simulink model "A1_DC_coupled_AC_output_grid_interface_DC_forming"  (R2022b)
settings: Solver=ode4  StartTime=0.0  StopTime=tend  FixedStep=ts  RelTol=1e-3
values from neighbouring files (symbols this model uses):
  C = 80000e-6    (= 0.08)    [A1_Parameters.m]
  C_bc_ESS = C_bc_ESS    (= 0.005)    [A1_Parameters.m]
  C_bc_PV = C_bc_PV    (= 0.005)    [A1_Parameters.m]
  C_bc_SC = C_bc_SC    (= 0.005)    [A1_Parameters.m]
  C_SC_set = C_SC * Vdc_SCunit^2/Vdc_SC^2    (= 0.617283950617)    [A1_Parameters.m]
  Cf = 0.08    [A1_Parameters.m]
  f0 = 60    [A1_Parameters.m]
  fc = 20    [A1_Parameters.m]
  fc1 = 1000    [A1_Parameters.m]
  fv = 100    [A1_Parameters.m]
  Idcbase = Sbase/Vdc_nom    (= 1250)    [A1_Parameters.m]
  J = [0 -1; 1 0]    [A1_Parameters.m]
  Ki_c = 500    [A1_Parameters.m]
  Ki_v = 500    [A1_Parameters.m]
  Ki_v1 = 1000    [A1_Parameters.m]
  Kp_c = 10    [A1_Parameters.m]
  Kp_v = 5    [A1_Parameters.m]
  Kp_v1 = 50    [A1_Parameters.m]
  L_bc_ESS = 4e-4    (= 0.0004)    [A1_Parameters.m]
  L_bc_PV = 4e-4    (= 0.0004)    [A1_Parameters.m]
  L_bc_SC = 4e-4    (= 0.0004)    [A1_Parameters.m]
  Lf = 0.10    (= 0.1)    [A1_Parameters.m]
  Pset_ESS = 0.0    (= 0)    [A1_Parameters.m]
  Pset_inv = Pset_PV + Pset_ESS + Pset_load    (= 0.4)    [A1_Parameters.m]
  Pset_load = -0.1    [A1_Parameters.m]
  Pset_PV = 0.5    [A1_Parameters.m]
  Pset_SC = 0.0    (= 0)    [A1_Parameters.m]
  Qset_inv = 0.0    (= 0)    [A1_Parameters.m]
  R_bc_ESS = 1e-3    (= 0.001)    [A1_Parameters.m]
  R_bc_PV = 1e-3    (= 0.001)    [A1_Parameters.m]
  R_bc_SC = 1e-3    (= 0.001)    [A1_Parameters.m]
  R_line_ESS = 1e-3    (= 0.001)    [A1_Parameters.m]
  R_line_PV = 1e-3    (= 0.001)    [A1_Parameters.m]
  R_line_SC = 1e-3    (= 0.001)    [A1_Parameters.m]
  Rf = 5e-4    (= 0.0005)    [A1_Parameters.m]
  Rg = 0.04 * 2    (= 0.08)    [A1_Parameters.m]
  Sbase = Stotal    (= 1000000)    [A1_Parameters.m]
  Stotal = 1e6    (= 1000000)    [A1_Parameters.m]
  tdist1 = 2    [A1_Parameters.m]
  tdist2 = 4    [A1_Parameters.m]
  tESSconnect = 0.1    [A1_Parameters.m]
  tPVconnect = 0.3    [A1_Parameters.m]
  ts = 5e-6    (= 5e-06)    [A1_Parameters.m]
  tSCconnect = 0.2    [A1_Parameters.m]
  V1 = 4160    [A1_Parameters.m]
  V2 = 400    [A1_Parameters.m]
  Vac_peak = Vac_nom*sqrt(2)/sqrt(3)    [A1_Parameters.m]
  Vdc_ESS = 480    [A1_Parameters.m]
  Vdc_nom = 800    [A1_Parameters.m]
  Vdc_PV = 480    [A1_Parameters.m]
  Vdc_PV0 = 464.3    [A1_Parameters.m]
  Vdc_SC = Vdc_SCunit * 180    (= 486)    [A1_Parameters.m]
  Vdc_SC0 = Vdc_SC    (= 486)    [A1_Parameters.m]
  Vset_inv = 1.05    [A1_Parameters.m]
  w0 = 2*pi*f0    (= 376.991118431)    [A1_Parameters.m]
  Zbase = Vbase^2/Sbase    (= 17.3056)    [A1_Parameters.m]
  Zg = 0.2 * 2    (= 0.4)    [A1_Parameters.m]
undefined symbols (not defined in the file or in its folder): Gf, Ilim, L_line_ESS, L_line_PV, Pnom, sps, Vnom
libraries: spsControlledVoltageSourceLib x15, spsSeriesRLCBranchLib x12, cstblocks x11, spsVoltageMeasurementLib x8, spsCurrentMeasurementLib x6, simulink_extras x5, spsGroundLib x5, spsThreePhaseVIMeasurementLib x4, spsBreakerLib x4, spsThreePhaseSeriesRLCBranchLib x4, spsThreePhaseTransformerTwoWindingsLib x3, spsPWMGeneratorDCDCLib x3
(part 1 of 2)
settings Model: Creator=josueduarte  LastModifiedBy=hxq19
settings DataIOCC: ReturnWorkspaceOutputs=off
settings DebuggingCC: AlgebraicLoopMsg=none
settings ModelReferenceCC: EnableRefExpFcnMdlSchedulingChecks=on

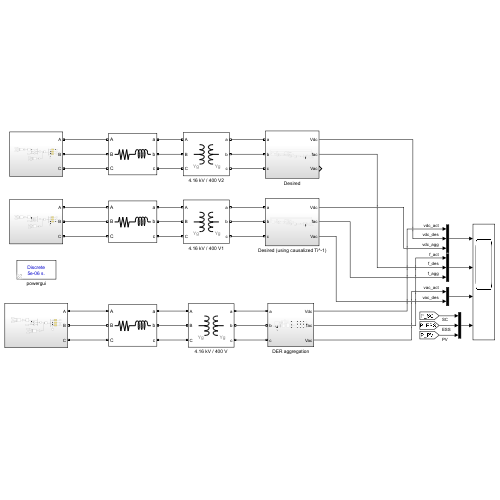
[thumbnail: Simulink's stored preview of the top-level diagram]
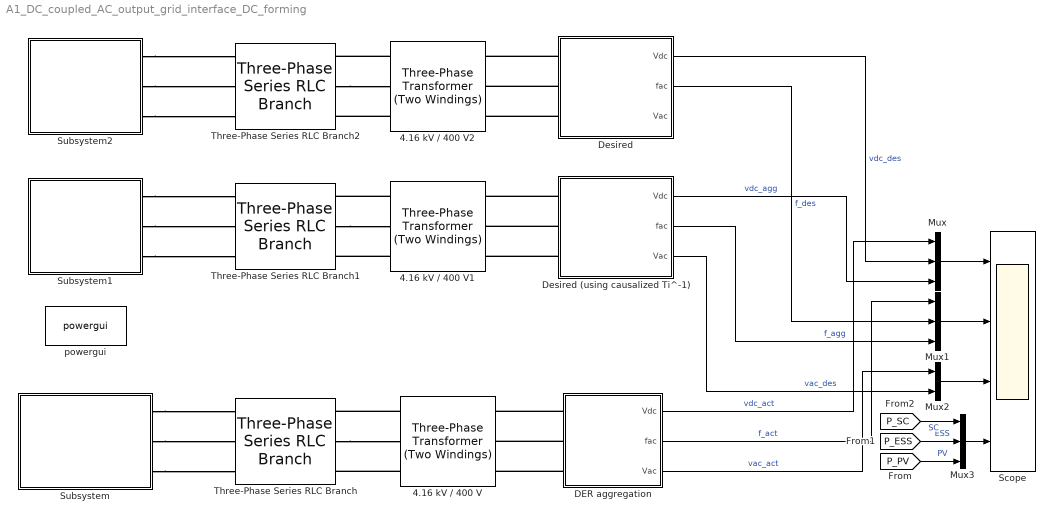
== system A1_DC_coupled_AC_output_grid_interface_DC_forming ==
  4.16 kV / 400 V : spsThreePhaseTransformerTwoWindingsLib/Three-Phase Transformer (Two Windings)  Winding1Connection=Yg  Winding2Connection=Yg  CoreType=Three single-phase transformers  SetSaturation=off  Hysteresis=off  DataFile='hysteresis'  SetInitialFlux=off  Measurements=None  UNITS=pu  NominalPower=[Stotal,f0]  Winding1=[ V1 , 0.001 , 0.03 ]  Winding2=[ V2 , 0.001 , 0.03 ]  Rm=500  Lm=inf  L0=0.5  Saturation=[ 0,0 ; 0.0024,1.2 ; 1.0,1.52 ]  InitialFluxes=[ 0.8 , -0.8 , 0.7 ]  BreakLoop=off  DiscreteSolver=Trapezoidal iterative  DataType=off  TransfoNumber=0
  4.16 kV / 400 V1 : spsThreePhaseTransformerTwoWindingsLib/Three-Phase Transformer (Two Windings)  Winding1Connection=Yg  Winding2Connection=Yg  CoreType=Three single-phase transformers  SetSaturation=off  Hysteresis=off  DataFile='hysteresis'  SetInitialFlux=off  Measurements=None  UNITS=pu  NominalPower=[Stotal,f0]  Winding1=[ V1 , 0.001 , 0.03 ]  Winding2=[ V2 , 0.001 , 0.03 ]  Rm=500  Lm=inf  L0=0.5  Saturation=[ 0,0 ; 0.0024,1.2 ; 1.0,1.52 ]  InitialFluxes=[ 0.8 , -0.8 , 0.7 ]  BreakLoop=off  DiscreteSolver=Trapezoidal iterative  DataType=off  TransfoNumber=0
  4.16 kV / 400 V2 : spsThreePhaseTransformerTwoWindingsLib/Three-Phase Transformer (Two Windings)  Winding1Connection=Yg  Winding2Connection=Yg  CoreType=Three single-phase transformers  SetSaturation=off  Hysteresis=off  DataFile='hysteresis'  SetInitialFlux=off  Measurements=None  UNITS=pu  NominalPower=[Stotal,f0]  Winding1=[ V1 , 0.001 , 0.03 ]  Winding2=[ V2 , 0.001 , 0.03 ]  Rm=500  Lm=inf  L0=0.5  Saturation=[ 0,0 ; 0.0024,1.2 ; 1.0,1.52 ]  InitialFluxes=[ 0.8 , -0.8 , 0.7 ]  BreakLoop=off  DiscreteSolver=Trapezoidal iterative  DataType=off  TransfoNumber=0
  DER aggregation : Subsystem
      settings: PortSchema="{\"entries\":[{\"content\":{\"sides\":[{\"content\":{\"connectorIds\":[\"Out1\",\"Out2\",\"Out3\"]},\"type\":\"ConnectorPlacement.EquallySpacedRectSide\",\"uuid\":\"b7b146c6-db8e-4a9c-9e78-599d288ba224\"},{\"content\":{\"connectorIds\":[\"RConn1\",\"RConn2\",\"RConn3\"],\"side\":\"RIGHT\"},\"type\":\"ConnectorPlacement.EquallySpacedRectSide\",\"uuid\":\"95d7d183-946c-4a3f-97eb-ffd2b4a90781\"},{\"content\":{\"connectorIds\":[],\"side\":\"TOP\"},\"type\":\"ConnectorPlacement.EquallySpacedRectSide\",\"uuid\":\"9b52036b-0c68-4ea6-b97f-d0d2327eba86\"}]},\"type\":\"ConnectorPlacement.EquallySpacedConnector\",\"uuid\":\"c5513f55-e830-4946-abb4-6597f92e93ee\"}],\"packageUris\":[\"http://schema.mathworks.com/mf0/Connector/R2020b\"],\"version\":\"1.0\"}"
  Desired : Subsystem
      settings: PortSchema="{\"entries\":[{\"content\":{\"sides\":[{\"content\":{\"connectorIds\":[\"Out1\",\"Out2\",\"Out3\"]},\"type\":\"ConnectorPlacement.EquallySpacedRectSide\",\"uuid\":\"d17645c7-cdec-4633-b3c6-cd15445995c3\"},{\"content\":{\"connectorIds\":[\"RConn1\",\"RConn2\",\"RConn3\"],\"side\":\"RIGHT\"},\"type\":\"ConnectorPlacement.EquallySpacedRectSide\",\"uuid\":\"25a3cf30-901e-4740-a075-3c8408526c60\"},{\"content\":{\"connectorIds\":[],\"side\":\"TOP\"},\"type\":\"ConnectorPlacement.EquallySpacedRectSide\",\"uuid\":\"8cde02ff-980e-4e20-bc67-22f4d69f4d72\"}]},\"type\":\"ConnectorPlacement.EquallySpacedConnector\",\"uuid\":\"2536287c-4269-40cd-b41b-6d4dfba348bd\"}],\"packageUris\":[\"http://schema.mathworks.com/mf0/Connector/R2020b\"],\"version\":\"1.0\"}"
  Desired (using causalized Ti^-1) : Subsystem
      settings: PortSchema="{\"entries\":[{\"content\":{\"sides\":[{\"content\":{\"connectorIds\":[\"Out1\",\"Out2\",\"Out3\"]},\"type\":\"ConnectorPlacement.EquallySpacedRectSide\",\"uuid\":\"d17645c7-cdec-4633-b3c6-cd15445995c3\"},{\"content\":{\"connectorIds\":[\"RConn1\",\"RConn2\",\"RConn3\"],\"side\":\"RIGHT\"},\"type\":\"ConnectorPlacement.EquallySpacedRectSide\",\"uuid\":\"25a3cf30-901e-4740-a075-3c8408526c60\"},{\"content\":{\"connectorIds\":[],\"side\":\"TOP\"},\"type\":\"ConnectorPlacement.EquallySpacedRectSide\",\"uuid\":\"8cde02ff-980e-4e20-bc67-22f4d69f4d72\"}]},\"type\":\"ConnectorPlacement.EquallySpacedConnector\",\"uuid\":\"2536287c-4269-40cd-b41b-6d4dfba348bd\"}],\"packageUris\":[\"http://schema.mathworks.com/mf0/Connector/R2020b\"],\"version\":\"1.0\"}"
  Mux : Mux  Inputs=3
  Mux1 : Mux  Inputs=3
  Mux2 : Mux  Inputs=2
  Mux3 : Mux  Inputs=3
  Scope : Scope  NumInputPorts=4
  Subsystem : Subsystem
  Subsystem1 : Subsystem
  Subsystem2 : Subsystem
  Three-Phase Series RLC Branch : spsThreePhaseSeriesRLCBranchLib/Three-Phase Series RLC Branch  LConnTagsString=A|B|C  RConnTagsString=A|B|C  BranchType=RL  Resistance=Rg*Zbase  Inductance=Zg*Zbase/w0  Capacitance=1e-6  Measurements=None
  Three-Phase Series RLC Branch1 : spsThreePhaseSeriesRLCBranchLib/Three-Phase Series RLC Branch  LConnTagsString=A|B|C  RConnTagsString=A|B|C  BranchType=RL  Resistance=Rg*Zbase  Inductance=Zg*Zbase/w0  Capacitance=1e-6  Measurements=None
  Three-Phase Series RLC Branch2 : spsThreePhaseSeriesRLCBranchLib/Three-Phase Series RLC Branch  LConnTagsString=A|B|C  RConnTagsString=A|B|C  BranchType=RL  Resistance=Rg*Zbase  Inductance=Zg*Zbase/w0  Capacitance=1e-6  Measurements=None
  powergui : spspowerguiLib/powergui  Priority=1  SimulationMode=Discrete  SampleTime=ts  frequency=60  Iterations=50  frequencyindice=0  Pbase=100e6  ErrMax=1e-4  UnitsV=kV  UnitsW=MW  buscounter=0  FunctionMessages=off  echomessages=off  EnableUseOfTLC=off  CurrentSourceSwitches=off  DisableSnubberDevices=off  DisableRonSwitches=off  DisableVfSwitches=off  DisplayEquations=off  AutomaticDiscreteSolvers=off  SolverType=Tustin/Backward Euler (TBE)  Interpol=off  ExternalGateDelay=off  methode=off  Ts=100  x0status=blocks  SPID=on  SwTol=0  HookPort=off  NonlinearTolerance=1e-4  nMaxIteration=100  ContinueOnMaxIteration=off  RestoreLinks=warning  ResistiveCurrentMeasurement=off  Frange=[0:2:500]  Ylog=off  Xlog=on  ShowGrid=off  save=off  variable=ZData  structure=0  ZoomFFT=off  StartTime=0.0  cycles=1  DisplayStyle=1  fundamental=60  FreqAxis=off  MaxFrequency=1000  frequencyindicesteady=1  RmsSteady=1  display=off
  wires:
  DER aggregation/3(Vac) -> Mux2/1  "vac_act"
  DER aggregation/2(fac) -> Mux1/1  "f_act"
  DER aggregation/1(Vdc) -> Mux/1  "vdc_act"
  Mux2/1 -> Scope/3
  Mux1/1 -> Scope/2
  Mux/1 -> Scope/1
  Desired (using causalized Ti^-1)/1(Vdc) -> Mux/3  "vdc_agg"
  Desired (using causalized Ti^-1)/2(fac) -> Mux1/3  "f_agg"
  Desired (using causalized Ti^-1)/3(Vac) -> Mux2/2  "vac_des"
  Mux3/1 -> Scope/4
  [P_ESS] -> Mux3/2  "ESS"
  Desired/1(Vdc) -> Mux/2  "vdc_des"
  Desired/2(fac) -> Mux1/2  "f_des"
  [P_PV] -> Mux3/3  "PV"
  [P_SC] -> Mux3/1  "SC"
  connections:
  Subsystem/RConn1 -- Three-Phase Series RLC Branch/LConn1
  Subsystem/RConn2 -- Three-Phase Series RLC Branch/LConn2
  Subsystem/RConn3 -- Three-Phase Series RLC Branch/LConn3
  4.16 kV / 400 V/LConn1 -- Three-Phase Series RLC Branch/RConn1
  Three-Phase Series RLC Branch/RConn2 -- 4.16 kV / 400 V/LConn2
  4.16 kV / 400 V/LConn3 -- Three-Phase Series RLC Branch/RConn3
  4.16 kV / 400 V1/LConn1 -- Three-Phase Series RLC Branch1/RConn1
  Subsystem1/RConn1 -- Three-Phase Series RLC Branch1/LConn1
  Subsystem1/RConn2 -- Three-Phase Series RLC Branch1/LConn2
  Subsystem1/RConn3 -- Three-Phase Series RLC Branch1/LConn3
  4.16 kV / 400 V1/LConn3 -- Three-Phase Series RLC Branch1/RConn3
  Three-Phase Series RLC Branch1/RConn2 -- 4.16 kV / 400 V1/LConn2
  Three-Phase Series RLC Branch2/RConn2 -- 4.16 kV / 400 V2/LConn2
  4.16 kV / 400 V2/LConn3 -- Three-Phase Series RLC Branch2/RConn3
  Subsystem2/RConn3 -- Three-Phase Series RLC Branch2/LConn3
  Subsystem2/RConn2 -- Three-Phase Series RLC Branch2/LConn2
  Subsystem2/RConn1 -- Three-Phase Series RLC Branch2/LConn1
  4.16 kV / 400 V2/LConn1 -- Three-Phase Series RLC Branch2/RConn1
  DER aggregation/RConn1 -- 4.16 kV / 400 V/RConn1
  DER aggregation/RConn2 -- 4.16 kV / 400 V/RConn2
  DER aggregation/RConn3 -- 4.16 kV / 400 V/RConn3
  Desired/RConn1 -- 4.16 kV / 400 V2/RConn1
  Desired/RConn2 -- 4.16 kV / 400 V2/RConn2
  Desired/RConn3 -- 4.16 kV / 400 V2/RConn3
  Desired (using causalized Ti^-1)/RConn1 -- 4.16 kV / 400 V1/RConn1
  Desired (using causalized Ti^-1)/RConn2 -- 4.16 kV / 400 V1/RConn2
  Desired (using causalized Ti^-1)/RConn3 -- 4.16 kV / 400 V1/RConn3

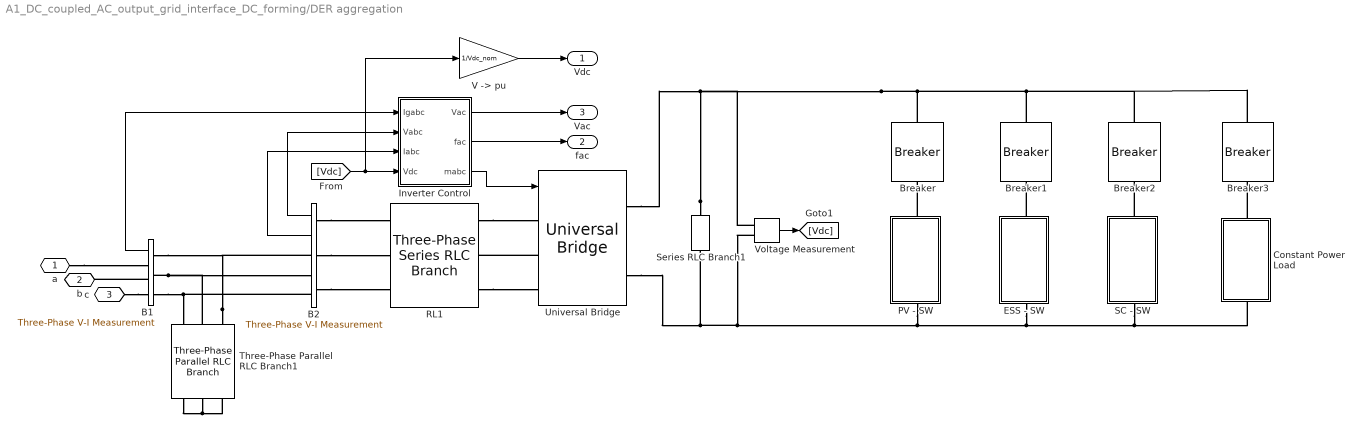
== system A1_DC_coupled_AC_output_grid_interface_DC_forming/DER aggregation ==
  B1 : spsThreePhaseVIMeasurementLib/Three-Phase V-I Measurement  VoltageMeasurement=no  SetLabelV=off  LabelV=Vabc_B1  Vpu=off  VpuLL=off  CurrentMeasurement=yes  SetLabelI=off  LabelI=Iabc_B1  Ipu=off  Pbase=100e6  Vbase=500e3  OutputType=Magnitude  PhasorSimulation=off  PSBequivalent=0
  B2 : spsThreePhaseVIMeasurementLib/Three-Phase V-I Measurement  VoltageMeasurement=phase-to-ground  SetLabelV=off  LabelV=Vabc_B1  Vpu=off  VpuLL=off  CurrentMeasurement=yes  SetLabelI=off  LabelI=Iabc_B1  Ipu=off  Pbase=100e6  Vbase=500e3  OutputType=Magnitude  PhasorSimulation=off  PSBequivalent=0
  Breaker : spsBreakerLib/Breaker  InitialState=0  SwitchingTimes=tPVconnect  External=off  BreakerResistance=1e-6  SnubberResistance=1e6  SnubberCapacitance=inf  Measurements=None  MoreParameters=on  NoBreakLoop=off
  Breaker1 : spsBreakerLib/Breaker  InitialState=0  SwitchingTimes=tESSconnect  External=off  BreakerResistance=1e-6  SnubberResistance=1e6  SnubberCapacitance=inf  Measurements=None  MoreParameters=on  NoBreakLoop=off
  Breaker2 : spsBreakerLib/Breaker  InitialState=0  SwitchingTimes=tSCconnect  External=off  BreakerResistance=1e-6  SnubberResistance=1e6  SnubberCapacitance=inf  Measurements=None  MoreParameters=on  NoBreakLoop=off
  Breaker3 : spsBreakerLib/Breaker  InitialState=0  SwitchingTimes=tLoadconnect  External=off  BreakerResistance=1e-6  SnubberResistance=1e6  SnubberCapacitance=inf  Measurements=None  MoreParameters=on  NoBreakLoop=off
  Constant Power Load : Subsystem
      settings: PortSchema="{\"entries\":[{\"content\":{\"sides\":[{\"content\":{\"connectorIds\":[]},\"type\":\"ConnectorPlacement.EquallySpacedRectSide\",\"uuid\":\"d64f8841-075a-4592-9721-07346c3eedde\"},{\"content\":{\"connectorIds\":[],\"side\":\"RIGHT\"},\"type\":\"ConnectorPlacement.EquallySpacedRectSide\",\"uuid\":\"f70d4421-2220-4657-8c99-8abb3184730b\"},{\"content\":{\"connectorIds\":[\"LConn1\"],\"side\":\"TOP\"},\"type\":\"ConnectorPlacement.EquallySpacedRectSide\",\"uuid\":\"2f586390-110d-4cc5-90f4-9aa5cf771f84\"},{\"content\":{\"connectorIds\":[\"RConn1\"],\"side\":\"BOTTOM\"},\"type\":\"ConnectorPlacement.EquallySpacedRectSide\",\"uuid\":\"57b4e366-61ab-45b5-95e6-2e46cf17a950\"}]},\"type\":\"ConnectorPlacement.EquallySpacedConnector\",\"uuid\":\"1143dd7b-038b-41e2-a355-4aaf746039e3\"}],\"packageUris\":[\"http://schema.mathworks.com/mf0/Connector/R2020b\"],\"version\":\"1.0\"}"
  ESS - SW : Subsystem
      settings: PortSchema="{\"entries\":[{\"content\":{\"sides\":[{\"content\":{\"connectorIds\":[]},\"type\":\"ConnectorPlacement.EquallySpacedRectSide\",\"uuid\":\"a366de01-415d-4fc7-8830-9a15956661b9\"},{\"content\":{\"connectorIds\":[],\"side\":\"RIGHT\"},\"type\":\"ConnectorPlacement.EquallySpacedRectSide\",\"uuid\":\"8598060f-9f02-4b93-be08-39bfe2a310b6\"},{\"content\":{\"connectorIds\":[\"LConn1\"],\"side\":\"TOP\"},\"type\":\"ConnectorPlacement.EquallySpacedRectSide\",\"uuid\":\"f1589895-78fb-4c72-b1f6-5b4e7ce7130b\"},{\"content\":{\"connectorIds\":[\"RConn1\"],\"side\":\"BOTTOM\"},\"type\":\"ConnectorPlacement.EquallySpacedRectSide\",\"uuid\":\"0a878aa3-6d51-479d-a764-f7fa1ccbaa9c\"}]},\"type\":\"ConnectorPlacement.EquallySpacedConnector\",\"uuid\":\"4d15ead3-9d78-44e1-8395-50a3f1c02350\"}],\"packageUris\":[\"http://schema.mathworks.com/mf0/Connector/R2020b\"],\"version\":\"1.0\"}"
  Inverter Control : Subsystem
  PV - SW : Subsystem
      settings: PortSchema="{\"entries\":[{\"content\":{\"sides\":[{\"content\":{\"connectorIds\":[]},\"type\":\"ConnectorPlacement.EquallySpacedRectSide\",\"uuid\":\"a366de01-415d-4fc7-8830-9a15956661b9\"},{\"content\":{\"connectorIds\":[],\"side\":\"RIGHT\"},\"type\":\"ConnectorPlacement.EquallySpacedRectSide\",\"uuid\":\"8598060f-9f02-4b93-be08-39bfe2a310b6\"},{\"content\":{\"connectorIds\":[\"LConn1\"],\"side\":\"TOP\"},\"type\":\"ConnectorPlacement.EquallySpacedRectSide\",\"uuid\":\"f1589895-78fb-4c72-b1f6-5b4e7ce7130b\"},{\"content\":{\"connectorIds\":[\"RConn1\"],\"side\":\"BOTTOM\"},\"type\":\"ConnectorPlacement.EquallySpacedRectSide\",\"uuid\":\"0a878aa3-6d51-479d-a764-f7fa1ccbaa9c\"}]},\"type\":\"ConnectorPlacement.EquallySpacedConnector\",\"uuid\":\"4d15ead3-9d78-44e1-8395-50a3f1c02350\"}],\"packageUris\":[\"http://schema.mathworks.com/mf0/Connector/R2020b\"],\"version\":\"1.0\"}"
  RL1 : spsThreePhaseSeriesRLCBranchLib/Three-Phase Series RLC Branch  LConnTagsString=A|B|C  RConnTagsString=A|B|C  BranchType=RL  Resistance=Rf*V2^2/(Sbase)  Inductance=Lf*V2^2/(Sbase)/(w0)  Capacitance=inf  Measurements=None
  SC - SW : Subsystem
      settings: PortSchema="{\"entries\":[{\"content\":{\"sides\":[{\"content\":{\"connectorIds\":[]},\"type\":\"ConnectorPlacement.EquallySpacedRectSide\",\"uuid\":\"a366de01-415d-4fc7-8830-9a15956661b9\"},{\"content\":{\"connectorIds\":[],\"side\":\"RIGHT\"},\"type\":\"ConnectorPlacement.EquallySpacedRectSide\",\"uuid\":\"8598060f-9f02-4b93-be08-39bfe2a310b6\"},{\"content\":{\"connectorIds\":[\"LConn1\"],\"side\":\"TOP\"},\"type\":\"ConnectorPlacement.EquallySpacedRectSide\",\"uuid\":\"f1589895-78fb-4c72-b1f6-5b4e7ce7130b\"},{\"content\":{\"connectorIds\":[\"RConn1\"],\"side\":\"BOTTOM\"},\"type\":\"ConnectorPlacement.EquallySpacedRectSide\",\"uuid\":\"0a878aa3-6d51-479d-a764-f7fa1ccbaa9c\"}]},\"type\":\"ConnectorPlacement.EquallySpacedConnector\",\"uuid\":\"4d15ead3-9d78-44e1-8395-50a3f1c02350\"}],\"packageUris\":[\"http://schema.mathworks.com/mf0/Connector/R2020b\"],\"version\":\"1.0\"}"
  Series RLC Branch1 : spsSeriesRLCBranchLib/Series RLC Branch  LConnTagsString=__new0  RConnTagsString=__new0  BranchType=C  Resistance=0.1  Inductance=3e-3  SetiL0=off  InitialCurrent=0  Capacitance=C  Setx0=on  InitialVoltage=Vdc_nom  Measurements=None
  Three-Phase Parallel RLC Branch1 : spsThreePhaseParallelRLCBranchLib/Three-Phase Parallel RLC Branch  LConnTagsString=A|B|C  RConnTagsString=A|B|C  BranchType=C  Resistance=1/Gf*Vnom^2/(Pnom)  Inductance=1e-3  Capacitance=Cf*(Sbase)/V2^2/(w0)  Measurements=None
  Universal Bridge : spsUniversalBridgeLib/Universal Bridge  Arms=3  SnubberResistance=1e5  SnubberCapacitance=inf  Device=IGBT / Diodes  Ron=1e-4  Lon=0  ForwardVoltages="[  0  0  ]"  ForwardVoltage=0  GTOparameters=[ 10e-6 , 20e-6 ]  IGBTparameters=[ 1e-6 , 2e-6 ]  Measurements=None  Measurements_2=None  converterType=Rectifier
  "V -> pu" : Gain  Gain=1/Vdc_nom
  Voltage Measurement : spsVoltageMeasurementLib/Voltage Measurement  PhasorSimulation=off  OutputType=Complex  PSBequivalent=0
  a : PMIOPort  Side=Right
  b : PMIOPort  Port=2  Side=Right
  c : PMIOPort  Port=3  Side=Right
  Vdc : Outport
  fac : Outport  Port=2
  Vac : Outport  Port=3
  wires:
  B2/2 -> Inverter Control/3(Iabc)
  "V -> pu"/1 -> Vdc/1
  [Vdc] -> Inverter Control/4(Vdc), "V -> pu"/1
  B2/1 -> Inverter Control/2(Vabc)
  B1/1 -> Inverter Control/1(Igabc)
  Inverter Control/3(mabc) -> Universal Bridge/1
  Inverter Control/2(fac) -> fac/1
  Inverter Control/1(Vac) -> Vac/1
  Voltage Measurement/1 -> [Vdc]
  connections:
  B1/RConn2 -- b/RConn1
  B2/LConn2 -- RL1/LConn2
  c/RConn1 -- B1/RConn3
  RL1/RConn1 -- Universal Bridge/LConn1
  RL1/RConn3 -- Universal Bridge/LConn3
  Universal Bridge/LConn2 -- RL1/RConn2
  B2/LConn3 -- RL1/LConn3
  a/RConn1 -- B1/RConn1
  B2/LConn1 -- RL1/LConn1
  B1/LConn2 -- B2/RConn2 -- Three-Phase Parallel RLC Branch1/LConn2
  B1/LConn3 -- B2/RConn3 -- Three-Phase Parallel RLC Branch1/LConn1
  Three-Phase Parallel RLC Branch1/RConn1 -- Three-Phase Parallel RLC Branch1/RConn3 -- Three-Phase Parallel RLC Branch1/RConn2
  Three-Phase Parallel RLC Branch1/LConn3 -- B2/RConn1 -- B1/LConn1
  SC - SW/LConn1 -- Breaker2/RConn1
  ESS - SW/LConn1 -- Breaker1/RConn1
  PV - SW/LConn1 -- Breaker/RConn1
  Series RLC Branch1/LConn1 -- Universal Bridge/RConn1 -- Breaker/LConn1 -- Breaker1/LConn1 -- Breaker3/LConn1 -- Breaker2/LConn1 -- Voltage Measurement/LConn1
  Voltage Measurement/LConn2 -- Constant Power Load/RConn1 -- SC - SW/RConn1 -- ESS - SW/RConn1 -- PV - SW/RConn1 -- Universal Bridge/RConn2 -- Series RLC Branch1/RConn1
  Constant Power Load/LConn1 -- Breaker3/RConn1

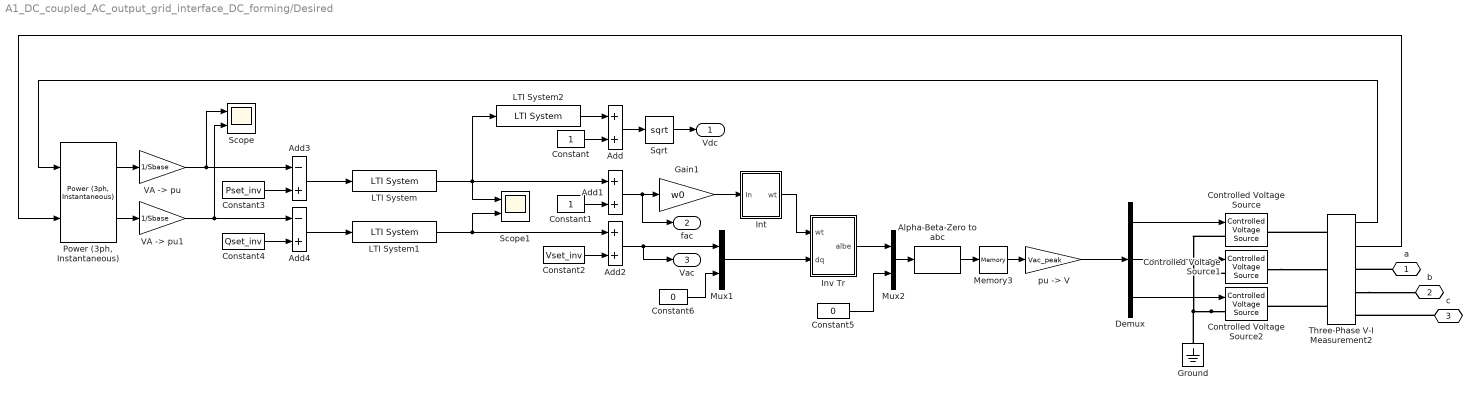
== system A1_DC_coupled_AC_output_grid_interface_DC_forming/Desired ==
  Add : Sum
  Add1 : Sum
  Add2 : Sum
  Add3 : Sum  Inputs=-+
  Add4 : Sum  Inputs=-+
  Alpha-Beta-Zero to abc : spsAlphaBetaZerotoabcLib/Alpha-Beta-Zero to abc
  Constant : Constant
  Constant1 : Constant
  Constant2 : Constant  Value=Vset_inv
  Constant3 : Constant  Value=Pset_inv
  Constant4 : Constant  Value=Qset_inv
  Constant5 : Constant  Value=0
  Constant6 : Constant  Value=0
  Controlled Voltage Source : spsControlledVoltageSourceLib/Controlled Voltage Source  Initialize=on  Source_Type=AC  Amplitude=0  Phase=0  Frequency=0  Measurements=None
  Controlled Voltage Source1 : spsControlledVoltageSourceLib/Controlled Voltage Source  Initialize=on  Source_Type=AC  Amplitude=0  Phase=0  Frequency=0  Measurements=None
  Controlled Voltage Source2 : spsControlledVoltageSourceLib/Controlled Voltage Source  Initialize=on  Source_Type=AC  Amplitude=0  Phase=0  Frequency=0  Measurements=None
  Demux : Demux  Outputs=3
  Gain1 : Gain  Gain=w0
  Ground : spsGroundLib/Ground  LConnTagsString=a
  Int : Subsystem
  Inv Tr : Subsystem
  LTI System : cstblocks/LTI System  sys=T_des_fp  IC=[]
  LTI System1 : cstblocks/LTI System  sys=T_des_vq  IC=[]
  LTI System2 : cstblocks/LTI System  sys=T_des_vdcf  IC=[]
  Memory3 : Memory
  Mux1 : Mux  Inputs=2
  Mux2 : Mux  Inputs=2
  "Power (3ph, Instantaneous)" : spsPower3phInstantaneousLib/Power (3ph, Instantaneous)
  Scope : Scope  NumInputPorts=2
  Scope1 : Scope  NumInputPorts=2
  Sqrt : Sqrt
  Three-Phase V-I Measurement2 : spsThreePhaseVIMeasurementLib/Three-Phase V-I Measurement  VoltageMeasurement=phase-to-ground  SetLabelV=off  LabelV=Vabc  Vpu=off  VpuLL=off  CurrentMeasurement=yes  SetLabelI=off  LabelI=Iabc  Ipu=off  Pbase=Sbase  Vbase=V2  OutputType=Complex  PhasorSimulation=off  PSBequivalent=0
  "VA -> pu" : Gain  Gain=1/Sbase
  "VA -> pu1" : Gain  Gain=1/Sbase
  "pu -> V" : Gain  Gain=Vac_peak
  a : PMIOPort  Side=Right
  b : PMIOPort  Port=2  Side=Right
  c : PMIOPort  Port=3  Side=Right
  Vdc : Outport
  fac : Outport  Port=2
  Vac : Outport  Port=3
  wires:
  Sqrt/1 -> Vdc/1
  Constant3/1 -> Add3/2
  LTI System2/1 -> Add/1
  Constant4/1 -> Add4/2
  "VA -> pu"/1 -> Scope/1, Add3/1
  Add/1 -> Sqrt/1
  "Power (3ph, Instantaneous)"/2 -> "VA -> pu1"/1
  "VA -> pu1"/1 -> Scope/2, Add4/1
  "Power (3ph, Instantaneous)"/1 -> "VA -> pu"/1
  Add2/1 -> Vac/1, Mux1/1
  Add4/1 -> LTI System1/1
  LTI System1/1 -> Scope1/2, Add2/1
  Constant1/1 -> Add1/2
  Add3/1 -> LTI System/1
  Constant/1 -> Add/2
  LTI System/1 -> Scope1/1, Add1/1, LTI System2/1
  Constant2/1 -> Add2/2
  Add1/1 -> fac/1, Gain1/1
  Mux2/1 -> Alpha-Beta-Zero to abc/1
  Alpha-Beta-Zero to abc/1 -> Memory3/1
  Memory3/1 -> "pu -> V"/1
  Mux1/1 -> Inv Tr/2(dq)
  Int/1(wt) -> Inv Tr/1(wt)
  Gain1/1 -> Int/1(In)
  Constant5/1 -> Mux2/2
  Inv Tr/1(albe) -> Mux2/1
  Constant6/1 -> Mux1/2
  Demux/1 -> Controlled Voltage Source/1
  Demux/2 -> Controlled Voltage Source1/1
  Demux/3 -> Controlled Voltage Source2/1
  "pu -> V"/1 -> Demux/1
  Three-Phase V-I Measurement2/1 -> "Power (3ph, Instantaneous)"/1
  Three-Phase V-I Measurement2/2 -> "Power (3ph, Instantaneous)"/2
  connections:
  Three-Phase V-I Measurement2/LConn3 -- Controlled Voltage Source2/RConn1
  Controlled Voltage Source1/RConn1 -- Three-Phase V-I Measurement2/LConn2
  Three-Phase V-I Measurement2/LConn1 -- Controlled Voltage Source/RConn1
  Controlled Voltage Source2/LConn1 -- Ground/LConn1 -- Controlled Voltage Source/LConn1 -- Controlled Voltage Source1/LConn1
  a/RConn1 -- Three-Phase V-I Measurement2/RConn1
  Three-Phase V-I Measurement2/RConn2 -- b/RConn1
  c/RConn1 -- Three-Phase V-I Measurement2/RConn3

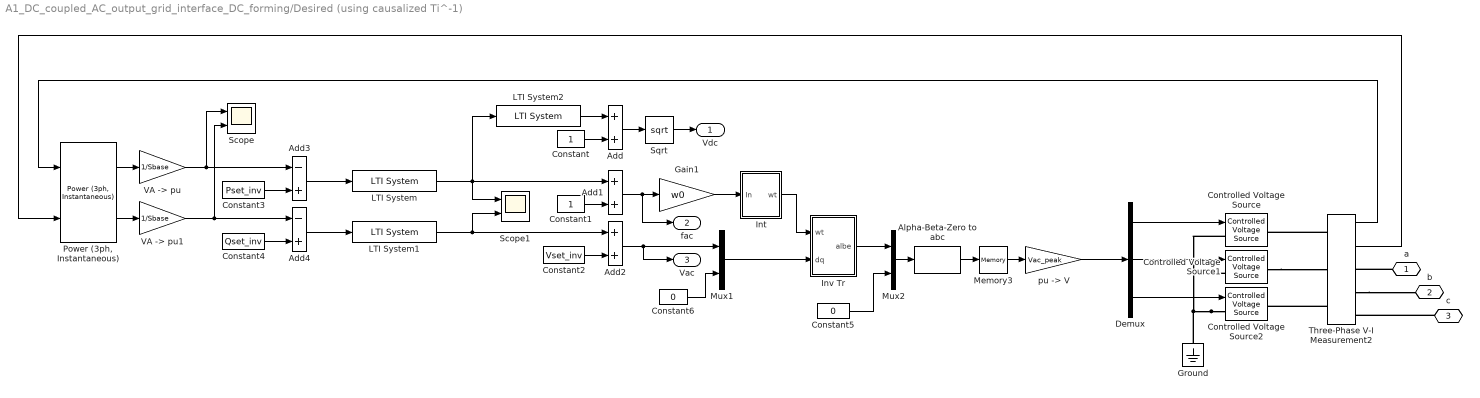
== system A1_DC_coupled_AC_output_grid_interface_DC_forming/Desired (using causalized Ti^-1) ==
  Add : Sum
  Add1 : Sum
  Add2 : Sum
  Add3 : Sum  Inputs=-+
  Add4 : Sum  Inputs=-+
  Alpha-Beta-Zero to abc : spsAlphaBetaZerotoabcLib/Alpha-Beta-Zero to abc
  Constant : Constant
  Constant1 : Constant
  Constant2 : Constant  Value=Vset_inv
  Constant3 : Constant  Value=Pset_inv
  Constant4 : Constant  Value=Qset_inv
  Constant5 : Constant  Value=0
  Constant6 : Constant  Value=0
  Controlled Voltage Source : spsControlledVoltageSourceLib/Controlled Voltage Source  Initialize=on  Source_Type=AC  Amplitude=0  Phase=0  Frequency=0  Measurements=None
  Controlled Voltage Source1 : spsControlledVoltageSourceLib/Controlled Voltage Source  Initialize=on  Source_Type=AC  Amplitude=0  Phase=0  Frequency=0  Measurements=None
  Controlled Voltage Source2 : spsControlledVoltageSourceLib/Controlled Voltage Source  Initialize=on  Source_Type=AC  Amplitude=0  Phase=0  Frequency=0  Measurements=None
  Demux : Demux  Outputs=3
  Gain1 : Gain  Gain=w0
  Ground : spsGroundLib/Ground  LConnTagsString=a
  Int : Subsystem
  Inv Tr : Subsystem
  LTI System : cstblocks/LTI System  sys=T_des_fp_agg_2  IC=[]
  LTI System1 : cstblocks/LTI System  sys=T_des_vq  IC=[]
  LTI System2 : cstblocks/LTI System  sys=T_des_vdcf  IC=[]
  Memory3 : Memory
  Mux1 : Mux  Inputs=2
  Mux2 : Mux  Inputs=2
  "Power (3ph, Instantaneous)" : spsPower3phInstantaneousLib/Power (3ph, Instantaneous)
  Scope : Scope  NumInputPorts=2
  Scope1 : Scope  NumInputPorts=2
  Sqrt : Sqrt
  Three-Phase V-I Measurement2 : spsThreePhaseVIMeasurementLib/Three-Phase V-I Measurement  VoltageMeasurement=phase-to-ground  SetLabelV=off  LabelV=Vabc  Vpu=off  VpuLL=off  CurrentMeasurement=yes  SetLabelI=off  LabelI=Iabc  Ipu=off  Pbase=Sbase  Vbase=V2  OutputType=Complex  PhasorSimulation=off  PSBequivalent=0
  "VA -> pu" : Gain  Gain=1/Sbase
  "VA -> pu1" : Gain  Gain=1/Sbase
  "pu -> V" : Gain  Gain=Vac_peak
  a : PMIOPort  Side=Right
  b : PMIOPort  Port=2  Side=Right
  c : PMIOPort  Port=3  Side=Right
  Vdc : Outport
  fac : Outport  Port=2
  Vac : Outport  Port=3
  wires:
  Sqrt/1 -> Vdc/1
  Constant3/1 -> Add3/2
  LTI System2/1 -> Add/1
  Constant4/1 -> Add4/2
  "VA -> pu"/1 -> Scope/1, Add3/1
  Add/1 -> Sqrt/1
  "Power (3ph, Instantaneous)"/2 -> "VA -> pu1"/1
  "VA -> pu1"/1 -> Scope/2, Add4/1
  "Power (3ph, Instantaneous)"/1 -> "VA -> pu"/1
  Add2/1 -> Vac/1, Mux1/1
  Add4/1 -> LTI System1/1
  LTI System1/1 -> Scope1/2, Add2/1
  Constant1/1 -> Add1/2
  Add3/1 -> LTI System/1
  Constant/1 -> Add/2
  LTI System/1 -> Scope1/1, Add1/1, LTI System2/1
  Constant2/1 -> Add2/2
  Add1/1 -> fac/1, Gain1/1
  Mux2/1 -> Alpha-Beta-Zero to abc/1
  Alpha-Beta-Zero to abc/1 -> Memory3/1
  Memory3/1 -> "pu -> V"/1
  Mux1/1 -> Inv Tr/2(dq)
  Int/1(wt) -> Inv Tr/1(wt)
  Gain1/1 -> Int/1(In)
  Constant5/1 -> Mux2/2
  Inv Tr/1(albe) -> Mux2/1
  Constant6/1 -> Mux1/2
  Demux/1 -> Controlled Voltage Source/1
  Demux/2 -> Controlled Voltage Source1/1
  Demux/3 -> Controlled Voltage Source2/1
  "pu -> V"/1 -> Demux/1
  Three-Phase V-I Measurement2/1 -> "Power (3ph, Instantaneous)"/1
  Three-Phase V-I Measurement2/2 -> "Power (3ph, Instantaneous)"/2
  connections:
  Three-Phase V-I Measurement2/LConn3 -- Controlled Voltage Source2/RConn1
  Controlled Voltage Source1/RConn1 -- Three-Phase V-I Measurement2/LConn2
  Three-Phase V-I Measurement2/LConn1 -- Controlled Voltage Source/RConn1
  Controlled Voltage Source2/LConn1 -- Ground/LConn1 -- Controlled Voltage Source/LConn1 -- Controlled Voltage Source1/LConn1
  a/RConn1 -- Three-Phase V-I Measurement2/RConn1
  Three-Phase V-I Measurement2/RConn2 -- b/RConn1
  c/RConn1 -- Three-Phase V-I Measurement2/RConn3

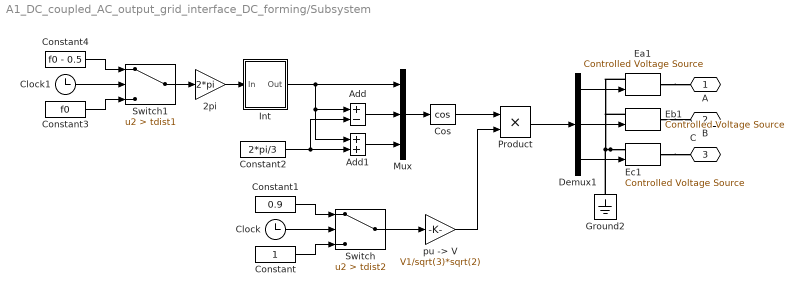
== system A1_DC_coupled_AC_output_grid_interface_DC_forming/Subsystem ==
  2pi : Gain  Gain=2*pi
  Add : Sum  Inputs=+-
  Add1 : Sum
  Clock : Clock
  Clock1 : Clock
  Constant : Constant
  Constant1 : Constant  Value=0.9
  Constant2 : Constant  Value=2*pi/3
  Constant3 : Constant  Value=f0
  Constant4 : Constant  Value=f0 - 0.5
  Cos : Trigonometry  Operator=cos
  Demux1 : Demux  Outputs=3
  Ea1 : spsControlledVoltageSourceLib/Controlled Voltage Source  Initialize=off  Source_Type=AC  Amplitude=0  Phase=0  Frequency=0  Measurements=None
  Eb1 : spsControlledVoltageSourceLib/Controlled Voltage Source  Initialize=off  Source_Type=AC  Amplitude=0  Phase=0  Frequency=0  Measurements=None
  Ec1 : spsControlledVoltageSourceLib/Controlled Voltage Source  Initialize=off  Source_Type=AC  Amplitude=0  Phase=0  Frequency=0  Measurements=None
  Ground2 : spsGroundLib/Ground  LConnTagsString=a
  Int : Subsystem
  Mux : Mux  Inputs=3
  Product : Product
  Switch : Switch  Criteria=u2 > Threshold  Threshold=tdist2  SaturateOnIntegerOverflow=off  InputSameDT=off
  Switch1 : Switch  Criteria=u2 > Threshold  Threshold=tdist1  SaturateOnIntegerOverflow=off  InputSameDT=off
  "pu -> V" : Gain  Gain=V1/sqrt(3)*sqrt(2)
  A : PMIOPort  Side=Right
  B : PMIOPort  Port=2  Side=Right
  C : PMIOPort  Port=3  Side=Right
  wires:
  Product/1 -> Demux1/1
  Demux1/1 -> Ea1/1
  Demux1/3 -> Ec1/1
  Demux1/2 -> Eb1/1
  Cos/1 -> Product/1
  "pu -> V"/1 -> Product/2
  Clock/1 -> Switch/2
  Constant/1 -> Switch/3
  Constant1/1 -> Switch/1
  Switch/1 -> "pu -> V"/1
  Mux/1 -> Cos/1
  Int/1(Out) -> Add/1, Add1/1, Mux/1
  Add/1 -> Mux/2
  Add1/1 -> Mux/3
  Constant2/1 -> Add/2, Add1/2
  Switch1/1 -> 2pi/1
  Constant4/1 -> Switch1/1
  Constant3/1 -> Switch1/3
  Clock1/1 -> Switch1/2
  2pi/1 -> Int/1(In)
  connections:
  Ea1/RConn1 -- A/RConn1
  Ec1/RConn1 -- C/RConn1
  Ec1/LConn1 -- Eb1/LConn1 -- Ea1/LConn1 -- Ground2/LConn1
  Eb1/RConn1 -- B/RConn1

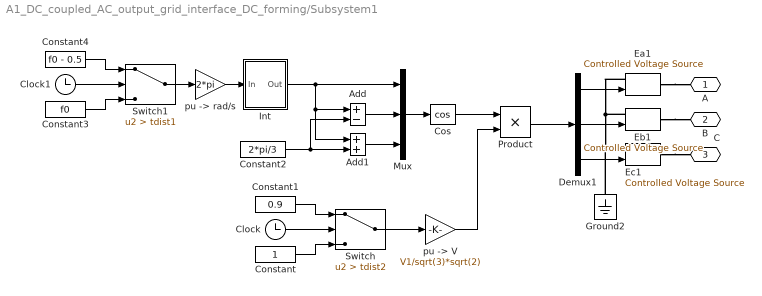
== system A1_DC_coupled_AC_output_grid_interface_DC_forming/Subsystem1 ==
  Add : Sum  Inputs=+-
  Add1 : Sum
  Clock : Clock
  Clock1 : Clock
  Constant : Constant
  Constant1 : Constant  Value=0.9
  Constant2 : Constant  Value=2*pi/3
  Constant3 : Constant  Value=f0
  Constant4 : Constant  Value=f0 - 0.5
  Cos : Trigonometry  Operator=cos
  Demux1 : Demux  Outputs=3
  Ea1 : spsControlledVoltageSourceLib/Controlled Voltage Source  Initialize=off  Source_Type=AC  Amplitude=0  Phase=0  Frequency=0  Measurements=None
  Eb1 : spsControlledVoltageSourceLib/Controlled Voltage Source  Initialize=off  Source_Type=AC  Amplitude=0  Phase=0  Frequency=0  Measurements=None
  Ec1 : spsControlledVoltageSourceLib/Controlled Voltage Source  Initialize=off  Source_Type=AC  Amplitude=0  Phase=0  Frequency=0  Measurements=None
  Ground2 : spsGroundLib/Ground  LConnTagsString=a
  Int : Subsystem
  Mux : Mux  Inputs=3
  Product : Product
  Switch : Switch  Criteria=u2 > Threshold  Threshold=tdist2  SaturateOnIntegerOverflow=off  InputSameDT=off
  Switch1 : Switch  Criteria=u2 > Threshold  Threshold=tdist1  SaturateOnIntegerOverflow=off  InputSameDT=off
  "pu -> V" : Gain  Gain=V1/sqrt(3)*sqrt(2)
  "pu -> rad/s" : Gain  Gain=2*pi
  A : PMIOPort  Side=Right
  B : PMIOPort  Port=2  Side=Right
  C : PMIOPort  Port=3  Side=Right
  wires:
  "pu -> rad/s"/1 -> Int/1(In)
  Clock1/1 -> Switch1/2
  Constant3/1 -> Switch1/3
  Constant4/1 -> Switch1/1
  Switch1/1 -> "pu -> rad/s"/1
  Constant2/1 -> Add1/2, Add/2
  Add1/1 -> Mux/3
  Add/1 -> Mux/2
  Int/1(Out) -> Mux/1, Add1/1, Add/1
  Mux/1 -> Cos/1
  Switch/1 -> "pu -> V"/1
  Constant1/1 -> Switch/1
  Constant/1 -> Switch/3
  Clock/1 -> Switch/2
  "pu -> V"/1 -> Product/2
  Cos/1 -> Product/1
  Demux1/2 -> Eb1/1
  Demux1/3 -> Ec1/1
  Demux1/1 -> Ea1/1
  Product/1 -> Demux1/1
  connections:
  Eb1/RConn1 -- B/RConn1
  Ea1/LConn1 -- Eb1/LConn1 -- Ec1/LConn1 -- Ground2/LConn1
  Ec1/RConn1 -- C/RConn1
  Ea1/RConn1 -- A/RConn1

== system A1_DC_coupled_AC_output_grid_interface_DC_forming/Subsystem2 ==
  Add : Sum  Inputs=+-
  Add1 : Sum
  Clock : Clock
  Clock1 : Clock
  Constant : Constant
  Constant1 : Constant  Value=0.9
  Constant2 : Constant  Value=2*pi/3
  Constant3 : Constant  Value=f0
  Constant4 : Constant  Value=f0 - 0.5
  Cos : Trigonometry  Operator=cos
  Demux1 : Demux  Outputs=3
  Ea1 : spsControlledVoltageSourceLib/Controlled Voltage Source  Initialize=off  Source_Type=AC  Amplitude=0  Phase=0  Frequency=0  Measurements=None
  Eb1 : spsControlledVoltageSourceLib/Controlled Voltage Source  Initialize=off  Source_Type=AC  Amplitude=0  Phase=0  Frequency=0  Measurements=None
  Ec1 : spsControlledVoltageSourceLib/Controlled Voltage Source  Initialize=off  Source_Type=AC  Amplitude=0  Phase=0  Frequency=0  Measurements=None
  Ground2 : spsGroundLib/Ground  LConnTagsString=a
  Int : Subsystem
  Mux : Mux  Inputs=3
  Product : Product
  Switch : Switch  Criteria=u2 > Threshold  Threshold=tdist2  SaturateOnIntegerOverflow=off  InputSameDT=off
  Switch1 : Switch  Criteria=u2 > Threshold  Threshold=tdist1  SaturateOnIntegerOverflow=off  InputSameDT=off
  "pu -> V" : Gain  Gain=V1/sqrt(3)*sqrt(2)
  "pu -> rad/s" : Gain  Gain=2*pi
  A : PMIOPort  Side=Right
  B : PMIOPort  Port=2  Side=Right
  C : PMIOPort  Port=3  Side=Right
  wires:
  Product/1 -> Demux1/1
  Demux1/1 -> Ea1/1
  Demux1/3 -> Ec1/1
  Demux1/2 -> Eb1/1
  Cos/1 -> Product/1
  "pu -> V"/1 -> Product/2
  Clock/1 -> Switch/2
  Constant/1 -> Switch/3
  Constant1/1 -> Switch/1
  Switch/1 -> "pu -> V"/1
  Mux/1 -> Cos/1
  Int/1(Out) -> Add/1, Add1/1, Mux/1
  Add/1 -> Mux/2
  Add1/1 -> Mux/3
  Constant2/1 -> Add/2, Add1/2
  Switch1/1 -> "pu -> rad/s"/1
  Constant4/1 -> Switch1/1
  Constant3/1 -> Switch1/3
  Clock1/1 -> Switch1/2
  "pu -> rad/s"/1 -> Int/1(In)
  connections:
  Ea1/RConn1 -- A/RConn1
  Ec1/RConn1 -- C/RConn1
  Ground2/LConn1 -- Ec1/LConn1 -- Eb1/LConn1 -- Ea1/LConn1
  Eb1/RConn1 -- B/RConn1

== system A1_DC_coupled_AC_output_grid_interface_DC_forming/DER aggregation/Constant Power Load ==
  Constant1 : Constant  Value=Pset_load
  Controlled Current Source2 : spsControlledCurrentSourceLib/Controlled Current Source  Initialize=on  Source_Type=DC  Amplitude=0  Phase=0  Frequency=0  Measurements=None
  Divide : Product  Inputs=/*
  Memory : Memory
  Saturation : Saturate  UpperLimit=1.5  LowerLimit=0.5
  Scope : Scope  NumInputPorts=2
  "V -> pu" : Gain  Gain=1/Vdc_nom
  Voltage Measurement : spsVoltageMeasurementLib/Voltage Measurement  PhasorSimulation=off  OutputType=Complex  PSBequivalent=0
  "pu -> A" : Gain  Gain=Idcbase
  + : PMIOPort  Side=Left
  - : PMIOPort  Port=2  Side=Right
  wires:
  "V -> pu"/1 -> Saturation/1
  Saturation/1 -> Scope/1, Divide/1
  Constant1/1 -> Divide/2
  "pu -> A"/1 -> Memory/1
  Divide/1 -> Scope/2, "pu -> A"/1
  [Vdc] -> "V -> pu"/1
  Voltage Measurement/1 -> [Vdc]
  Memory/1 -> Controlled Current Source2/1
  connections:
  Controlled Current Source2/RConn1 -- Voltage Measurement/LConn1 -- +/RConn1
  Controlled Current Source2/LConn1 -- Voltage Measurement/LConn2 -- -/RConn1

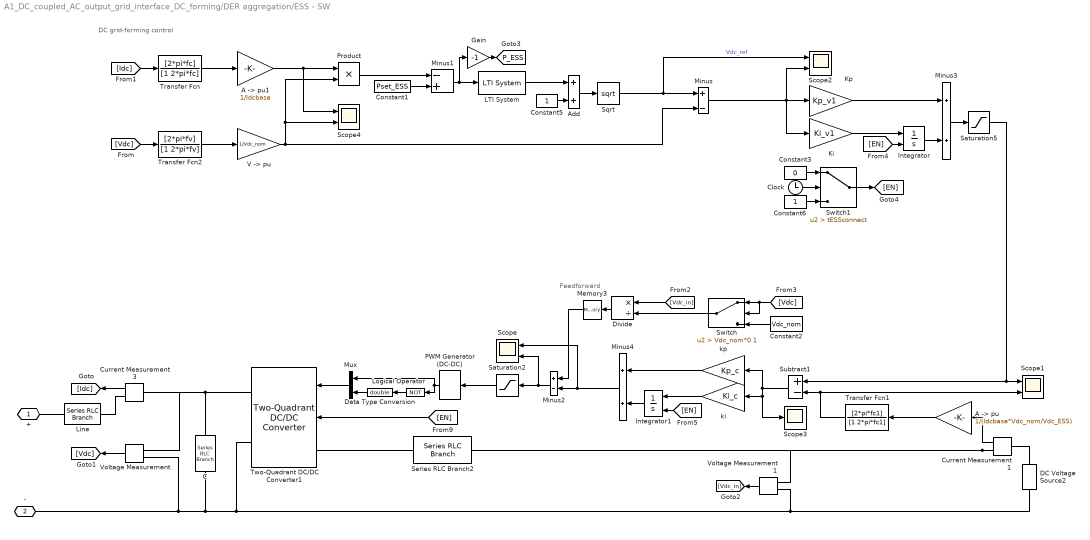
== system A1_DC_coupled_AC_output_grid_interface_DC_forming/DER aggregation/ESS - SW ==
  note: Feedforward
  note: DC grid-forming control
  "A -> pu" : Gain  Gain=1/(Idcbase*Vdc_nom/Vdc_ESS)
  "A -> pu1" : Gain  Gain=1/Idcbase
  Add : Sum
  C : spsSeriesRLCBranchLib/Series RLC Branch  LConnTagsString=__new0  RConnTagsString=__new0  BranchType=C  Resistance=0.001  Inductance=L_line_PV  SetiL0=off  InitialCurrent=0  Capacitance=C_bc_ESS  Setx0=on  InitialVoltage=Vdc_nom  Measurements=None
  Clock : Clock
  Constant1 : Constant  Value=Pset_ESS
  Constant2 : Constant  Value=Vdc_nom
  Constant3 : Constant  Value=0
  Constant5 : Constant
  Constant6 : Constant
  Current Measurement1 : spsCurrentMeasurementLib/Current Measurement  PhasorSimulation=off  OutputType=Complex  PSBequivalent=0
  Current Measurement3 : spsCurrentMeasurementLib/Current Measurement  PhasorSimulation=off  OutputType=Complex  PSBequivalent=0
  DC Voltage Source2 : spsDCVoltageSourceLib/DC Voltage Source  Amplitude=Vdc_ESS  Measurements=None
  Data Type Conversion : DataTypeConversion  OutDataTypeStr=double  SaturateOnIntegerOverflow=off  RndMeth=Floor
  Divide : Product  Inputs=*/
  Gain : Gain  Gain=-1
  Integrator : Integrator  ExternalReset=level hold  UpperSaturationLimit=1.5  LowerSaturationLimit=-0.5
  Integrator1 : Integrator  ExternalReset=level hold  LimitOutput=on  UpperSaturationLimit=1  LowerSaturationLimit=-1
  Ki : Gain  Gain=Ki_v1
  Kp : Gain  Gain=Kp_v1
  LTI System : cstblocks/LTI System  sys=T_inv_ESS  IC=[]
  Line : spsSeriesRLCBranchLib/Series RLC Branch  LConnTagsString=__new0  RConnTagsString=__new0  BranchType=R  Resistance=R_line_ESS  Inductance=L_line_ESS  SetiL0=off  InitialCurrent=0  Capacitance=1e-6  Setx0=off  InitialVoltage=0  Measurements=None
  Logical Operator : Logic  Operator=NOT  AllPortsSameDT=off  OutDataTypeStr=boolean
  Memory3 : Memory
  Minus : Sum  Inputs=+-
  Minus1 : Sum  Inputs=-+
  Minus2 : Sum  Inputs=+-
  Minus3 : Sum
  Minus4 : Sum
  Mux : Mux  Inputs=2
  PWM Generator (DC-DC) : spsPWMGeneratorDCDCLib/PWM Generator (DC-DC)  Fsw=fw  Ts=0
  Product : Product
  Saturation2 : Saturate  UpperLimit=1  LowerLimit=0
  Saturation5 : Saturate  UpperLimit=1.0  LowerLimit=-1.0
  Scope{,1..2,4} (4 alike) : Scope  NumInputPorts=2
  Scope3 : Scope
  Series RLC Branch2 : spsSeriesRLCBranchLib/Series RLC Branch  LConnTagsString=__new0  RConnTagsString=__new0  BranchType=RL  Resistance=R_bc_ESS  Inductance=L_bc_ESS  SetiL0=off  InitialCurrent=Pset_ESS*Idcbase*Vdc_nom/Vdc_PV  Capacitance=1e-6  Setx0=off  InitialVoltage=0  Measurements=None
  Sqrt : Sqrt
  Subtract1 : Sum  Inputs=+-
  Switch : Switch  Criteria=u2 > Threshold  Threshold=Vdc_nom*0.1  SaturateOnIntegerOverflow=off  InputSameDT=off
  Switch1 : Switch  Criteria=u2 > Threshold  Threshold=tESSconnect  SaturateOnIntegerOverflow=off  InputSameDT=off
  Transfer Fcn : TransferFcn  Numerator=[2*pi*fc]  Denominator=[1 2*pi*fc]
  Transfer Fcn1 : TransferFcn  Numerator=[2*pi*fc1]  Denominator=[1 2*pi*fc1]
  Transfer Fcn2 : TransferFcn  Numerator=[2*pi*fv]  Denominator=[1 2*pi*fv]
  Two-Quadrant DC/DC Converter1 : spsTwoQuadrantDCDCConverterLib/Two-Quadrant DC//DC Converter  ModelType=Switching devices  Ron=1e-4  Rs=1e6  Cs=inf  Vforward=[0,0]  Ron_Diode=1e-3  Rs_Diode=1e6  Cs_Diode=inf  Vf_Diode=1e-3  Rs_CurrentSource=inf  Ron_ACsource=1e-3
      settings: LibrarySourceBlock=|
      | sps_lib/Power Electronics/Two-Quadrant
      | DC//DC Converter
  "V -> pu" : Gain  Gain=1/Vdc_nom
  Voltage Measurement : spsVoltageMeasurementLib/Voltage Measurement  PhasorSimulation=off  OutputType=Complex  PSBequivalent=0
  Voltage Measurement1 : spsVoltageMeasurementLib/Voltage Measurement  PhasorSimulation=off  OutputType=Complex  PSBequivalent=0
  ki : Gain  Gain=Ki_c
  kp : Gain  Gain=Kp_c
  + : PMIOPort  Side=Left
  - : PMIOPort  Port=2  Side=Right
  tag scope: P_ESS=global
  wires:
  Transfer Fcn2/1 -> "V -> pu"/1
  Transfer Fcn/1 -> "A -> pu1"/1
  Minus2/1 -> Scope/2, Saturation2/1
  Minus/1 -> Scope2/2, Ki/1, Kp/1
  Minus4/1 -> Minus2/2, Scope/1
  [Vdc] -> Transfer Fcn2/1
  "A -> pu1"/1 -> Product/1, Scope4/1
  "V -> pu"/1 -> Scope4/2, Product/2, Minus/2
  Memory3/1 -> Minus2/1
  [EN] -> Integrator1/2
  [EN] -> Integrator/2
  Constant6/1 -> Switch1/3
  Constant3/1 -> Switch1/1
  Switch1/1 -> [EN]
  Clock/1 -> Switch1/2
  Subtract1/1 -> ki/1, Scope3/1, kp/1
  ki/1 -> Integrator1/1
  Integrator1/1 -> Minus4/2
  kp/1 -> Minus4/1
  Kp/1 -> Minus3/1
  Integrator/1 -> Minus3/2
  Ki/1 -> Integrator/1
  Saturation2/1 -> PWM Generator (DC-DC)/1
  Saturation5/1 -> Scope1/1, Subtract1/1
  Minus3/1 -> Saturation5/1
  [Vdc] -> Switch/1, Switch/2
  Voltage Measurement1/1 -> [Vdc_in]
  Divide/1 -> Memory3/1
  [Vdc_in] -> Divide/1
  Constant2/1 -> Switch/3
  Switch/1 -> Divide/2
  Sqrt/1 -> Scope2/1, Minus/1  "Vdc_ref"
  Add/1 -> Sqrt/1
  Constant5/1 -> Add/2
  LTI System/1 -> Add/1
  Minus1/1 -> Gain/1, LTI System/1
  Product/1 -> Minus1/1
  Transfer Fcn1/1 -> Subtract1/2, Scope1/2
  Current Measurement1/1 -> "A -> pu"/1
  [EN] -> Two-Quadrant DC/DC Converter1/2
  Constant1/1 -> Minus1/2
  Current Measurement3/1 -> [Idc]
  Voltage Measurement/1 -> [Vdc]
  [Idc] -> Transfer Fcn/1
  "A -> pu"/1 -> Transfer Fcn1/1
  Gain/1 -> [P_ESS]
  Mux/1 -> Two-Quadrant DC/DC Converter1/1
  PWM Generator (DC-DC)/1 -> Mux/1, Logical Operator/1
  Logical Operator/1 -> Data Type Conversion/1
  Data Type Conversion/1 -> Mux/2
  connections:
  Line/LConn1 -- +/RConn1
  C/LConn1 -- Two-Quadrant DC/DC Converter1/RConn1 -- Voltage Measurement/LConn1 -- Current Measurement3/LConn1
  Current Measurement3/RConn1 -- Line/RConn1
  Current Measurement1/RConn1 -- Voltage Measurement1/LConn1 -- Series RLC Branch2/RConn1
  DC Voltage Source2/RConn1 -- Current Measurement1/LConn1
  Two-Quadrant DC/DC Converter1/LConn1 -- Series RLC Branch2/LConn1
  Voltage Measurement/LConn2 -- -/RConn1 -- C/RConn1 -- Two-Quadrant DC/DC Converter1/RConn2 -- Voltage Measurement1/LConn2 -- DC Voltage Source2/LConn1

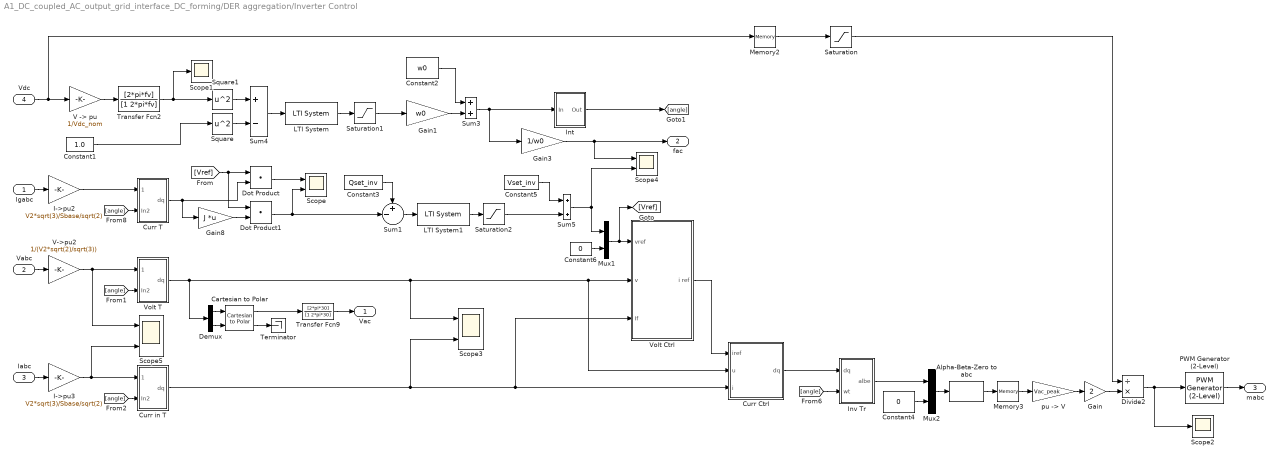
== system A1_DC_coupled_AC_output_grid_interface_DC_forming/DER aggregation/Inverter Control ==
  Igabc : Inport
  Vabc : Inport  Port=2
  Iabc : Inport  Port=3
  Vdc : Inport  Port=4
  Alpha-Beta-Zero to abc : spsAlphaBetaZerotoabcLib/Alpha-Beta-Zero to abc
  Cartesian to Polar : simulink_extras/Transformations/Cartesian to Polar
  Constant1 : Constant  Value=1.0
  Constant2 : Constant  Value=w0
  Constant3 : Constant  Value=Qset_inv
  Constant4 : Constant  Value=0
  Constant5 : Constant  Value=Vset_inv
  Constant6 : Constant  Value=0
  Curr Ctrl : Subsystem
  Curr T : Subsystem
  Curr in T : Subsystem
  Demux : Demux  Outputs=2
  Divide2 : Product  Inputs=/*
  Dot Product : DotProduct  OutDataTypeStr=Inherit: Inherit via internal rule
  Dot Product1 : DotProduct  OutDataTypeStr=Inherit: Inherit via internal rule
  Gain : Gain  Gain=2
  Gain1 : Gain  Gain=w0
  Gain3 : Gain  Gain=1/w0
  Gain8 : Gain  Gain=J  Multiplication=Matrix(K*u)
  I->pu2 : Gain  Gain=V2*sqrt(3)/Sbase/sqrt(2)  SaturateOnIntegerOverflow=on  OutDataTypeStr=Inherit: Same as input  ParamDataTypeStr=Inherit: Same as input
  I->pu3 : Gain  Gain=V2*sqrt(3)/Sbase/sqrt(2)  SaturateOnIntegerOverflow=on  OutDataTypeStr=Inherit: Same as input  ParamDataTypeStr=Inherit: Same as input
  Int : Subsystem
  Inv Tr : Subsystem
  LTI System : cstblocks/LTI System  sys=T_des_fvdc  IC=[]
  LTI System1 : cstblocks/LTI System  sys=T_des_vq  IC=[]
  Memory2 : Memory
  Memory3 : Memory
  Mux1 : Mux  Inputs=2
  Mux2 : Mux  Inputs=2
  PWM Generator (2-Level) : spsPWMGenerator2LevelLib/PWM Generator (2-Level)  ModulatorType=Three-phase bridge (6 pulses)  ModulatorMode=Unsynchronized  Fc=fw  Pc=90  nF=27  MinMax="[ -1  1 ]"  SamplingTechnique=Natural  ModulatingSignals=off  m=0.8  Freq=60  Phase=0  Ts=0  ShowCarrierOutport=off
  Saturation : Saturate  UpperLimit=Vdc_nom*1.1  LowerLimit=Vdc_nom*0.9
  Saturation1 : Saturate  UpperLimit=0.1  LowerLimit=-0.1
  Saturation2 : Saturate
  Scope{,3..5} (4 alike) : Scope  NumInputPorts=2
  Scope1 : Scope
  Scope2 : Scope
  Square : Math  Operator=square
  Square1 : Math  Operator=square
  Sum1 : Sum  Inputs=+-|
  Sum3 : Sum
  Sum4 : Sum  Inputs=+-
  Sum5 : Sum
  Terminator : Terminator
  Transfer Fcn2 : TransferFcn  Numerator=[2*pi*fv]  Denominator=[1 2*pi*fv]
  Transfer Fcn9 : TransferFcn  Numerator=[2*pi*30]  Denominator=[1 2*pi*30]
  "V -> pu" : Gain  Gain=1/Vdc_nom
  V->pu2 : Gain  Gain=1/(V2*sqrt(2)/sqrt(3))  SaturateOnIntegerOverflow=on  OutDataTypeStr=Inherit: Same as input  ParamDataTypeStr=Inherit: Same as input
  Volt Ctrl : Subsystem
  Volt T : Subsystem
  "pu -> V" : Gain  Gain=Vac_peak
  Vac : Outport
  fac : Outport  Port=2
  mabc : Outport  Port=3
  wires:
  Transfer Fcn9/1 -> Vac/1
  Memory3/1 -> "pu -> V"/1
  Curr Ctrl/1(dq) -> Inv Tr/1(dq)
  Mux1/1 -> Volt Ctrl/1(vref), [Vref]
  Constant6/1 -> Mux1/2
  Sum5/1 -> Mux1/1, Scope4/2
  Cartesian to Polar/1 -> Transfer Fcn9/1
  Cartesian to Polar/2 -> Terminator/1
  Demux/1 -> Cartesian to Polar/1
  Demux/2 -> Cartesian to Polar/2
  Int/1(Out) -> [angle]
  Inv Tr/1(albe) -> Mux2/1
  [angle] -> Inv Tr/2(wt)
  Volt Ctrl/1(i ref) -> Curr Ctrl/1(iref)
  Curr in T/1(dq) -> Curr Ctrl/3(i), Volt Ctrl/3(If), Scope3/2
  Volt T/1(dq) -> Scope3/1, Volt Ctrl/2(v), Curr Ctrl/2("u "), Demux/1
  Gain8/1 -> Dot Product1/2
  Curr T/1(dq) -> Gain8/1, Dot Product/2
  [Vref] -> Dot Product1/1, Dot Product/1
  [angle] -> Curr in T/2(In2)
  I->pu3/1 -> Curr in T/1(abc), Scope5/2
  V->pu2/1 -> Volt T/1(abc), Scope5/1
  [angle] -> Volt T/2(In2)
  [angle] -> Curr T/2(In2)
  I->pu2/1 -> Curr T/1(abc)
  Iabc/1 -> I->pu3/1
  PWM Generator (2-Level)/1 -> mabc/1
  Transfer Fcn2/1 -> Square1/1, Scope1/1
  Saturation1/1 -> Gain1/1
  Memory2/1 -> Saturation/1
  "V -> pu"/1 -> Transfer Fcn2/1
  Vdc/1 -> Memory2/1, "V -> pu"/1
  Saturation/1 -> Divide2/1
  Saturation2/1 -> Sum5/2
  LTI System/1 -> Saturation1/1
  Gain3/1 -> fac/1, Scope4/1
  Square1/1 -> Sum4/1
  Square/1 -> Sum4/2
  Constant3/1 -> Sum1/1
  Sum1/1 -> LTI System1/1
  Divide2/1 -> PWM Generator (2-Level)/1, Scope2/1
  "pu -> V"/1 -> Gain/1
  Dot Product1/1 -> Sum1/2, Scope/2
  Dot Product/1 -> Scope/1
  Constant1/1 -> Square/1
  Constant5/1 -> Sum5/1
  Mux2/1 -> Alpha-Beta-Zero to abc/1
  Gain1/1 -> Sum3/2
  Constant4/1 -> Mux2/2
  Sum4/1 -> LTI System/1
  LTI System1/1 -> Saturation2/1
  Constant2/1 -> Sum3/1
  Alpha-Beta-Zero to abc/1 -> Memory3/1
  Sum3/1 -> Gain3/1, Int/1(In)
  Gain/1 -> Divide2/2
  Vabc/1 -> V->pu2/1
  Igabc/1 -> I->pu2/1
